simulink model "motor_model"  (R2023a)
settings: Solver=VariableStepAuto  StartTime=0.0  StopTime=10  MaxStep=1e-3  RelTol=1e-3
values from neighbouring files (symbols this model uses):
  Kphi = 1.6    [motorValues.m]
  TL = 20    [motorValues.m]
  Va = 200    [motorValues.m]
settings Model: Creator=EMRIX  LastModifiedBy=EMRIX

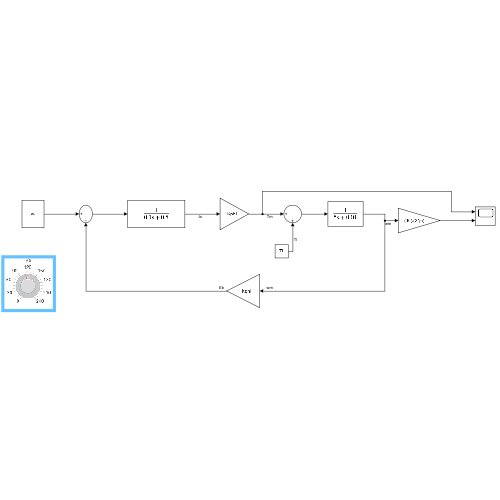
[thumbnail: Simulink's stored preview of the top-level diagram]
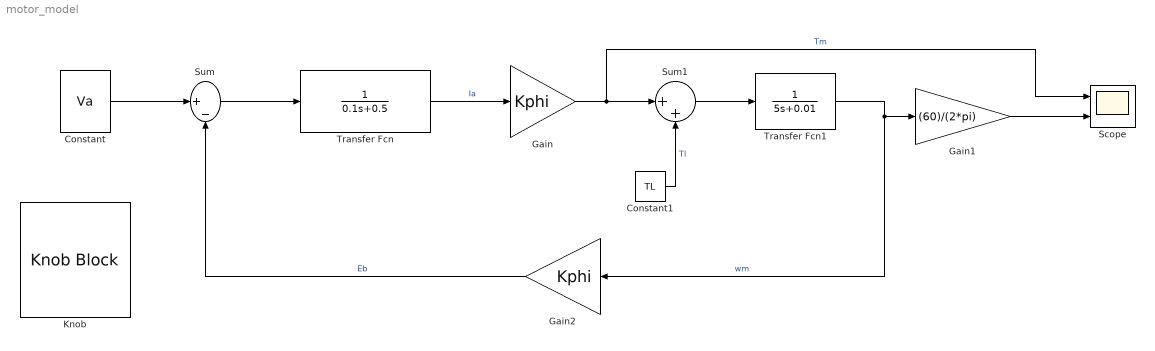
== system motor_model ==
  Constant : Constant  Value=Va
  Constant1 : Constant  Value=TL
  Gain : Gain  Gain=Kphi
  Gain1 : Gain  Gain=(60)/(2*pi)
  Gain2 : Gain  Gain=Kphi
  Knob : KnobBlock  ScaleMax=240
  Scope : Scope  NumInputPorts=2
  Sum : Sum  Inputs=|+-
  Sum1 : Sum  Inputs=|++
  Transfer Fcn : TransferFcn  Denominator=[0.1 0.5]
  Transfer Fcn1 : TransferFcn  Denominator=[5 0.01]
  wires:
  Constant/1 -> Sum/1
  Transfer Fcn1/1 -> Gain2/1, Gain1/1  "wm"
  Sum/1 -> Transfer Fcn/1
  Transfer Fcn/1 -> Gain/1  "Ia"
  Gain/1 -> Scope/1, Sum1/1  "Tm"
  Constant1/1 -> Sum1/2  "Tl"
  Sum1/1 -> Transfer Fcn1/1
  Gain2/1 -> Sum/2  "Eb"
  Gain1/1 -> Scope/2
